simulink model "SimulinkUnrealController"  (R2025b)
settings: Solver=FixedStepDiscrete  StartTime=0.0  StopTime=inf  RelTol=1e-3
model workspace (MAT data in the model file):
  patternLocation = [100 -60 0 0 0 0]
values from neighbouring files (symbols this model uses):
  ddxFilter = zeros(1080,1920)    [initVariables.m]
  ddyFilter = zeros(1080,1920)    [initVariables.m]
undefined symbols (not defined in the file or in its folder): Sim3dSensor
libraries: sim3dcameralib x3, sim3dlib x3, visionsinks x3
settings Model: Creator=Liam  LastModifiedBy=Liam
settings OptimizationCC: DefaultParameterBehavior=Inlined  EnhancedBackFolding=on  PassReuseOutputArgsAs=Individual arguments  ZeroExternalMemoryAtStartup=off  ZeroInternalMemoryAtStartup=off  OptimizeBlockOrder=speed  DifferentSizesBufferReuse=on  OptimizationCustomize=off  EfficientTunableParamExpr=on
settings DebuggingCC: ParameterTunabilityLossMsg=error
settings SFSimCC: MATLABDynamicMemAlloc=off
settings RTWCC: SystemTargetFile=ert.tlc  GenCodeOnly=on  TemplateMakefile=ert_default_tmf  TargetLang=C++  Description=Embedded Coder
settings CodeAppCC: ForceParamTrailComments=on  IgnoreCustomStorageClasses=off  OperatorAnnotations=on  SimulinkDataObjDesc=on  SFDataObjDesc=on  InsertBlockDesc=on
settings ERTTargetCC: RootIOFormat=Structure reference  ERTCustomFileTemplate=example_file_process.tlc  TargetLangStandard=C++11 (ISO)  GenerateSampleERTMain=on  CodeInterfacePackaging=C++ class  SubcomponentCodeInterfacePackaging=C++ class

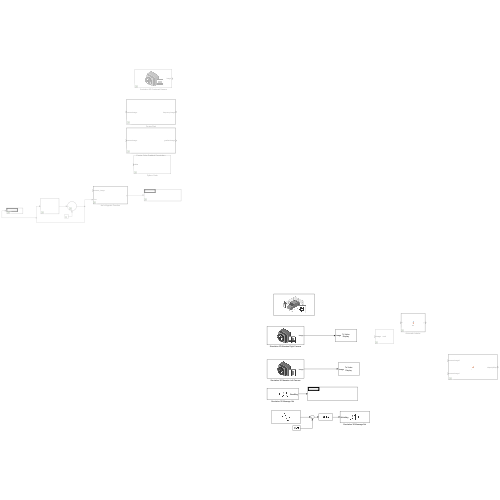
[thumbnail: Simulink's stored preview of the top-level diagram]
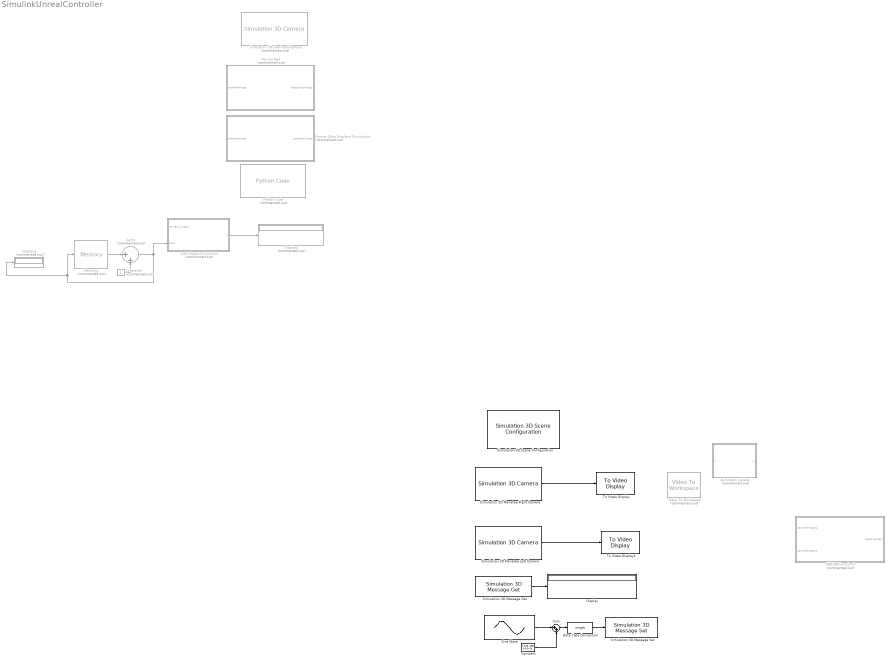
== system SimulinkUnrealController ==
  Automatic Labeler : MATLAB Function  Commented=on  TreatAsAtomicUnit=on
  Constant : Constant  Value=[-140 -450 0 0 0 -0]  VectorParams1D=off  OutDataTypeStr=single
  Constant5 : Constant  Commented=on
  Data Type Conversion : DataTypeConversion  OutDataTypeStr=single  SaturateOnIntegerOverflow=off  RndMeth=Floor
  Display : Display
  Display3 : Display  Commented=on
  Display4 : Display  Commented=on
  Fourier Color Gradient Convolution : MATLAB Function  Commented=on  TreatAsAtomicUnit=on
  Fourier Red : MATLAB Function  Commented=on  TreatAsAtomicUnit=on
  Joe's Keypoint Function : MATLAB Function  Commented=on  TreatAsAtomicUnit=on
  MATLAB Function3 : MATLAB Function  Commented=on  TreatAsAtomicUnit=on
  Memory2 : Memory  Commented=on
  Python Code : PythonCode  Commented=on
  Simulation 3D Manatee Left Camera : sim3dcameralib/Simulation 3D Camera  Priority=1  sensorTag=Sim3dSensor�  sensorId=1  sensorName=Sim3dSensor�  vehTagList={'Scene Origin'}  vehTag=Scene Origin  CoordinateSystem=Default  mountLoc=Origin  offsetFlag=on  tmountOffset=[40, -12.5, 15]/100  extTmount=off  rmountOffset=[0, 0, 0]  extRmount=off  FocalLength=[2.97 / 0.0028, 2.97 / 0.0028]  OpticalCenter=[960, 540]  ImageSize=[1080, 1920]  RadialDistortion=[0,0]  TangentialDistortion=[0, 0]  SensorSkew=0  VisualizeFieldOfView=off  FieldOfViewRange=61  DepthOutportEnabled=off  SemanticOutportEnabled=off  TransformOutportEnabled=off  SampleTime=-1  mountPoint=[0.4 -0.125 0.15]  mountOrientation=[0 0 0]  aMode=5  ID=1
      settings: LibrarySourceBlock=sl3dlib/Simulation 3D/Sensors/Simulation 3D Camera
  Simulation 3D Manatee Right Camera : sim3dcameralib/Simulation 3D Camera  Priority=1  sensorTag=Sim3dSensor�  sensorId=2  sensorName=Sim3dSensor�  vehTagList={'Scene Origin'}  vehTag=Scene Origin  CoordinateSystem=Default  mountLoc=Origin  offsetFlag=on  tmountOffset=[40, 12.5, 15]/100  extTmount=off  rmountOffset=[0, 0, 0]  extRmount=off  FocalLength=[2.97 / 0.0028, 2.97 / 0.0028]  OpticalCenter=[960, 540]  ImageSize=[1080, 1920]  RadialDistortion=[0,0]  TangentialDistortion=[0, 0]  SensorSkew=0  VisualizeFieldOfView=off  FieldOfViewRange=61  DepthOutportEnabled=off  SemanticOutportEnabled=off  TransformOutportEnabled=off  SampleTime=-1  mountPoint=[0.4 0.125 0.15]  mountOrientation=[0 0 0]  aMode=5  ID=2
      settings: LibrarySourceBlock=sl3dlib/Simulation 3D/Sensors/Simulation 3D Camera
  Simulation 3D Message Get : sim3dlib/Simulation 3D Message Get  Priority=1  SigName=ManateePoseGet  DataType=single  MsgSize=[1 6]  Ts=-1  aMode=0
      settings: LibrarySourceBlock=aerolibsim3d/Simulation 3D Message Get
  Simulation 3D Message Set : sim3dlib/Simulation 3D Message Set  Priority=-1  SigName=ManateePoseSet  Ts=-1  aMode=0
      settings: LibrarySourceBlock=aerolibsim3d/Simulation 3D Message Set
  Simulation 3D Overhead Camera : sim3dcameralib/Simulation 3D Camera  Priority=1  Commented=on  sensorTag=Sim3dSensor�  sensorId=3  sensorName=Sim3dSensor�  vehTagList={'Scene Origin'}  vehTag=Scene Origin  CoordinateSystem=Default  mountLoc=Origin  offsetFlag=on  tmountOffset=[-355, -565, 435]/100  extTmount=off  rmountOffset=[0, -35, 0]*pi/180  extRmount=off  FocalLength=[2.97 / 0.0028, 2.97 / 0.0028]  OpticalCenter=[960, 540]  ImageSize=[1080, 1920]  RadialDistortion=[0,0]  TangentialDistortion=[0, 0]  SensorSkew=0  VisualizeFieldOfView=off  FieldOfViewRange=61  DepthOutportEnabled=off  SemanticOutportEnabled=off  TransformOutportEnabled=off  SampleTime=-1  mountPoint=[-3.55 -5.65 4.35]  mountOrientation=[0 -0.610865238198015 0]  aMode=5  ID=3
      settings: LibrarySourceBlock=sl3dlib/Simulation 3D/Sensors/Simulation 3D Camera
  Simulation 3D Scene Configuration : sim3dlib/Simulation 3D Scene Configuration  Priority=0  ProjectFormat=Unreal Editor  SceneDesc=Straight road  ProjectName=C:\Program Files\MATLAB\R2025b\toolbox\shared\sim3d_projects\automotive_project_windows\UE\WindowsNoEditor\VehicleSimulation.exe  ScenePath=/Game/Maps/HwStrght  UEProjPath=C:\Users\Liam\OneDrive\Documents\GitHub\Vision_Sim\Unreal\UnrealProjects\SimulinkCoSimulation\EllingtonPoolSim\EllingtonPoolSim.uproject  EnableOpenDRIVE=off  vehTagList={'Custom';'Scene Origin'}  vehTag=Scene Origin  AttachedCameraRelativeTranslation=[0 0 0]  FreeCameraDefaultInitialTranslation=[-6, 0, 2]  AttachedCameraRelativeRotation=[0 0 0]  FreeCameraDefaultInitialRotation=[0, -15, 0]  ViewpointName=Custom  FreeCameraInitialTranslation=[0, 0, 0]  ViewpointTranslation=[0 0 0]  FreeCameraInitialRotation=[0, 0, 0]  ViewpointRotation=[0 0 0]  OpVisEn=off  Ts=1/60  EnableWindow=on  EnableRemoteAccess=off  EnableWeather=off  SunAzimuth=90  SunAltitude=40.0  EnableGeospatialSun=off  Latitude=0  Longitude=0  Date=2023-01-01  Time=10:30:00  GeoTimeZone=-5.0  SunDaylightSaving=off  wind=1  clouds=10  EnableVolumetricClouds=off  CloudCoverage=0  CloudAltitude=6  fog=0  rain=0  RaindropsEffect=off  SnowDensity=0  EnableGeospatial=off  TilesetSource=Earth terrain  UseTrueOrigin=off  OriginHeight=200  OriginLatitude=40.744652  OriginLongitude=-73.988864  MapStyle=Aerial  AdditionalAssetIDs=[]  UseAdvancedSunSky=off  SolarTime=11  TimeZone=-5  Day=21  Month=9  Year=2022  UseDaylightSavingTime=on  DSTStartDay=10  DSTStartMonth=3  DSTEndDay=3  DSTEndMonth=11  DSTSwitchHour=2  sensorTag=MainCamera1  sensorId=1  sensorName=MainCamera1  mountLoc=Origin  offsetFlag=off  tmountOffset=[0, 0, 0]  rmountOffset=[0, 0, 0]  HorizontalResolution=1280  VerticalResolution=720  HorizontalFOV=60  mountPoint=[0 0 0]  mountOrientation=[0 0 0]  aMode=3  ID=1  GeoTrigger=Inactive  ViewNameList={'Custom'}  ViewTranslationList={'[0 0 0]'}  ViewRotationList={'[0 0 0]'}
      settings: LibrarySourceBlock=drivingsim3d/Simulation 3D Scene Configuration
  Sine Wave : Sin  Amplitude=[0 100 0 30 3 20]  Frequency=[1.1,0.4,0.3,2,1,0.6]  SampleTime=0
  Sum : Sum  Inputs=|++
  Sum3 : Sum  Commented=on  Inputs=|++
  To Video Display : visionsinks/To Video Display  windowSizeMode=Normal  openAtMdlStart=on  fullScreen=off  videoWindowX=536805376  videoWindowY=536805376  saveWindowSize=off  videoWindowWidth=1920  videoWindowHeight=1080  inputColorFormat=RGB  inputType=Obsolete  imagePorts=One multidimensional signal  OutputDevice=On-screen video monitor  dataOrg=Column-major  isWindowOpen=off
  To Video Display1 : visionsinks/To Video Display  windowSizeMode=Normal  openAtMdlStart=on  fullScreen=off  videoWindowX=536805376  videoWindowY=536805376  saveWindowSize=off  videoWindowWidth=1920  videoWindowHeight=1080  inputColorFormat=RGB  inputType=Obsolete  imagePorts=One multidimensional signal  OutputDevice=On-screen video monitor  dataOrg=Column-major  isWindowOpen=off
  Video To Workspace : visionsinks/Video To Workspace  Commented=on  VariableName=vout  NumInputs=1  DataLimit=10  DecimationFactor=1  LogFi=off  InPortLabels=R|G|B
  wires:
  Simulation 3D Manatee Left Camera/1 -> To Video Display1/1
  Sine Wave/1 -> Sum/1
  Sum/1 -> Data Type Conversion/1
  Simulation 3D Message Get/1 -> Display/1
  Data Type Conversion/1 -> Simulation 3D Message Set/1
  Constant/1 -> Sum/2
  Constant5/1 -> Sum3/2
  Memory2/1 -> Sum3/1
  Sum3/1 -> Joe's Keypoint Function/2(time), Display3/1, Memory2/1
  Joe's Keypoint Function/1(y) -> Display4/1
  Simulation 3D Manatee Right Camera/1 -> To Video Display/1

== matlab function SimulinkUnrealController/Fourier Red ==
  data: frequencyImage output; cameraImage input
function frequencyImage = fcn(cameraImage)

redImage = cameraImage(:,:,1);

redImage = double(redImage) / 510.0;
F = fft2(redImage);
F = fftshift(F);
absF = abs(F);
logabsF = log(absF);

frequencyImage = logabsF;

== matlab function SimulinkUnrealController/Fourier Color Gradient Convolution ==
  data: gradientImage output; cameraImage input; ddxFilter parameter; ddyFilter parameter
function gradientImage = fcn(cameraImage, ddxFilter, ddyFilter)

redImage = cameraImage(:,:,1);

redImage = double(redImage) / 255.0;
redImageF = fft2(redImage);

ddxRedImageF = redImageF.*ddxFilter;
ddyRedImageF = redImageF.*ddyFilter;

ddxRedImage = abs(ifft2(ddxRedImageF));
ddyRedImage = abs(ifft2(ddyRedImageF));

greenImage = cameraImage(:,:,2);

greenImage = double(greenImage) / 255.0;
greenImageF = fft2(greenImage);

ddxGreenImageF = greenImageF.*ddxFilter;
ddyGreenImageF = greenImageF.*ddyFilter;

ddxGreenImage = abs(ifft2(ddxGreenImageF));
ddyGreenImage = abs(ifft2(ddyGreenImageF));

blueImage = cameraImage(:,:,3);

blueImage = double(blueImage) / 255.0;
blueImageF = fft2(blueImage);

ddxBlueImageF = blueImageF.*ddxFilter;
ddyBlueImageF = blueImageF.*ddyFilter;

ddxBlueImage = abs(ifft2(ddxBlueImageF));
ddyBlueImage = abs(ifft2(ddyBlueImageF));

gradientImage = zeros(1080, 1920);
for l = 1:1080
    for k = 1:1920
        gradientAbs = sqrt(ddxRedImage(l,k)^2 + ddyRedImage(l,k)^2 + ddxGreenImage(l,k)^2 + ddyGreenImage(l,k)^2 + ddxBlueImage(l,k)^2 + ddyBlueImage(l,k)^2);
        gradientImage(l,k) = gradientAbs;
    end
end

gradientImage = gradientImage / 20;

== matlab function SimulinkUnrealController/MATLAB Function3 ==
  data: cameraImage2 input; disparityMap output; cameraImage1 input
function disparityMap = fcn(cameraImage2, cameraImage1)

grayImage1 = im2gray(cameraImage1);
grayImage2 = im2gray(cameraImage2);

%edgeImage1 = edge(grayImage1, 'sobel');
%edgeImage2 = edge(grayImage2, 'sobel');

%[Gx1,Gy1] = imgradientxy(grayImage1,'sobel');
%[Gx2,Gy2] = imgradientxy(grayImage2,'sobel');

%gradientImage1 = sqrt(Gx1.^2 + Gy1.^2) / 800;
%gradientImage2 = sqrt(Gx2.^2 + Gy2.^2) / 800;
disparityRange = [8 128];
disparityMap = disparitySGM(grayImage1, grayImage2, "DisparityRange", disparityRange, "UniquenessThreshold", 30) / 96;




%grayImage1 = imgaussfilt(grayImage1,2);
%grayImage2 = imgaussfilt(grayImage2,2);

== matlab function SimulinkUnrealController/Automatic Labeler ==
  data: u input; y output
function y = fcn(u)

y = getWorldToImage(u, 'left');

disp(y);

== matlab function SimulinkUnrealController/Joe's Keypoint Function ==
  data: camera_image input; y output; time input
function y = fcn(camera_image, time)
coder.extrinsic('py.inference.predict')

result = py.inference.predict(camera_image);
y = zeros(4,2);
resultSize = zeros(1, 2);
resultSize = size(result);
if  resultSize == [4, 2]
    y = double(result);
end
